simulink model "Quadrotor"  (R2022b)
settings: Solver=FixedStepAuto  StartTime=0.0  StopTime=1000  FixedStep=0.0005  RelTol=1e-3
model workspace (MAT data in the model file):
  b = 0.000142
  g = 9.8
  m = 1
undefined symbols (not defined in the file): Pitch, Roll, X, Y, Yaw, Z
libraries: simulink x12, slpidlib x9, sharedtransform x1, uavutilslib x1, aerolibanim x1
(part 3 of 3)

== system Quadrotor/Attitude Loop(LADRC)/LADRC/TD ==
  v0 : Inport
  Constant : Constant  Value=r
  Constant1 : Constant  Value=0.05
  Gain : Gain  Gain=h
  Gain1 : Gain  Gain=h
  MATLAB Function : MATLAB Function  TreatAsAtomicUnit=on
  Sum : Sum  Inputs=+-|
  Sum1 : Sum  Inputs=++|
  Sum2 : Sum  Inputs=++|
  Unit Delay : UnitDelay  SampleTime=-1  HasFrameUpgradeWarning=on
  Unit Delay1 : UnitDelay  SampleTime=-1  HasFrameUpgradeWarning=on
  v1 : Outport
  v2 : Outport  Port=2
  wires:
  v0/1 -> Sum/2
  Unit Delay/1 -> Sum1/1, Sum/1  "v1(k"
  Unit Delay1/1 -> Sum2/1, MATLAB Function/2(v1), Gain/1  "v2(k)"
  Gain/1 -> Sum1/2
  Sum1/1 -> v1/1, Unit Delay/1  "v1(k+1)"
  Gain1/1 -> Sum2/2
  Sum2/1 -> v2/1, Unit Delay1/1  "v2(k+1)"
  MATLAB Function/1(y) -> Gain1/1
  Constant/1 -> MATLAB Function/3(r)
  Sum/1 -> MATLAB Function/1(delta)

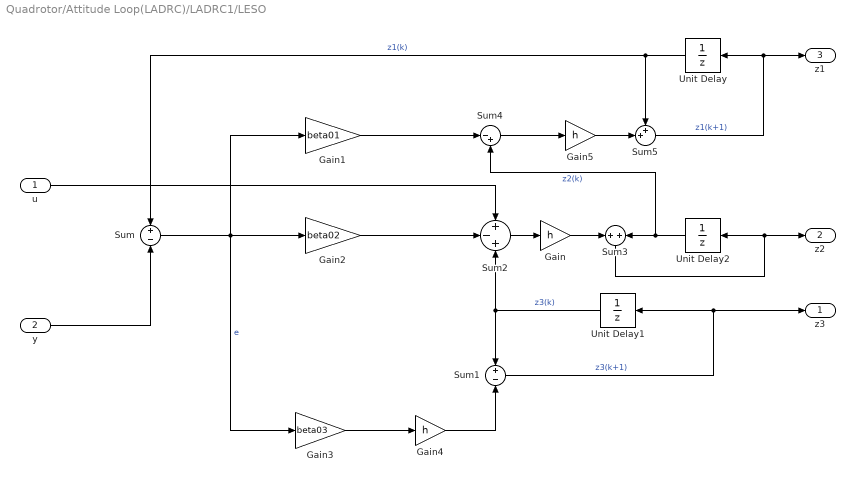
== system Quadrotor/Attitude Loop(LADRC)/LADRC1/LESO ==
  u : Inport
  y : Inport  Port=2
  Gain : Gain  Gain=h
  Gain1 : Gain  Gain=beta01
  Gain2 : Gain  Gain=beta02
  Gain3 : Gain  Gain=beta03
  Gain4 : Gain  Gain=h
  Gain5 : Gain  Gain=h
  Sum : Sum  Inputs=+|-
  Sum1 : Sum  Inputs=+-
  Sum2 : Sum  Inputs=+-+
  Sum3 : Sum
  Sum4 : Sum  Inputs=|-+
  Sum5 : Sum  Inputs=++|
  Unit Delay : UnitDelay  SampleTime=-1  HasFrameUpgradeWarning=on
  Unit Delay1 : UnitDelay  SampleTime=-1  HasFrameUpgradeWarning=on
  Unit Delay2 : UnitDelay  SampleTime=-1  HasFrameUpgradeWarning=on
  z3 : Outport
  z2 : Outport  Port=2
  z1 : Outport  Port=3
  wires:
  y/1 -> Sum/2
  Unit Delay/1 -> Sum/1, Sum5/1  "z1(k)"
  Unit Delay1/1 -> Sum2/3, Sum1/1  "z3(k)"
  Sum/1 -> Gain3/1, Gain1/1, Gain2/1  "e"
  Gain3/1 -> Gain4/1
  Gain4/1 -> Sum1/2
  Sum1/1 -> z3/1, Unit Delay1/1  "z3(k+1)"
  Gain2/1 -> Sum2/2
  Sum2/1 -> Gain/1
  Gain/1 -> Sum3/1
  Unit Delay2/1 -> Sum4/2, Sum3/2  "z2(k)"
  Sum3/1 -> Unit Delay2/1, z2/1
  Gain1/1 -> Sum4/1
  Sum4/1 -> Gain5/1
  Gain5/1 -> Sum5/2
  Sum5/1 -> Unit Delay/1, z1/1  "z1(k+1)"
  u/1 -> Sum2/1

== system Quadrotor/Attitude Loop(LADRC)/LADRC1/LSEF ==
  e1 : Inport
  e2 : Inport  Port=2
  Sum : Sum  Inputs=+-
  kp1 : Gain  Gain=kp1
  kp2 : Gain  Gain=kp2
  u0 : Outport
  wires:
  e1/1 -> kp1/1
  e2/1 -> kp2/1
  kp1/1 -> Sum/1
  kp2/1 -> Sum/2
  Sum/1 -> u0/1

== system Quadrotor/Attitude Loop(LADRC)/P&R/Pitch_LADRC ==
  v0 : Inport
  y : Inport  Port=2
  LESO : Subsystem
      settings: PortSchema="{\"entries\":[{\"content\":{\"sides\":[{\"content\":{\"connectorIds\":[]},\"type\":\"ConnectorPlacement.EquallySpacedRectSide\",\"uuid\":\"29853f4c-4dde-4de5-ade1-1dc0b5f537cd\"},{\"content\":{\"connectorIds\":[\"Out1\",\"Out2\",\"Out3\"],\"side\":\"RIGHT\"},\"type\":\"ConnectorPlacement.EquallySpacedRectSide\",\"uuid\":\"f82e0ac0-07eb-4296-b691-afdbd004b121\"},{\"content\":{\"connectorIds\":[\"In1\"],\"side\":\"TOP\"},\"type\":\"ConnectorPlacement.EquallySpacedRectSide\",\"uuid\":\"058c0543-22b7-4f39-8eab-a4fe87266d7e\"},{\"content\":{\"connectorIds\":[\"In2\"],\"side\":\"BOTTOM\"},\"type\":\"ConnectorPlacement.EquallySpacedRectSide\",\"uuid\":\"5206ee30-69dc-4d41-920c-ca25503196a3\"}]},\"type\":\"ConnectorPlacement.EquallySpacedConnector\",\"uuid\":\"8c454db7-eb5f-43d2-ac3f-1394779a05da\"}],\"packageUris\":[\"http://schema.mathworks.com/mf0/Connector/19700101\"],\"version\":\"1.0\"}"
  LSEF : Subsystem
  Sum : Sum  Inputs=|+-
  Sum1 : Sum  Inputs=|+-
  Sum2 : Sum  Inputs=|+-
  TD : Subsystem
  b1 : Gain  Gain=b
  b2 : Gain  Gain=1/b
  u : Outport
  wires:
  LESO/3(z1) -> Sum/2  "z1"
  LSEF/1(u0) -> Sum2/1
  Sum/1 -> LSEF/1(e1)  "e1"
  LESO/1(z3) -> Sum2/2
  Sum2/1 -> b2/1  "e1"
  b2/1 -> b1/1, u/1
  y/1 -> LESO/2(y)
  TD/1(v1) -> Sum/1
  v0/1 -> TD/1(v0)
  TD/2(v2) -> Sum1/1
  Sum1/1 -> LSEF/2(e2)  "e2"
  LESO/2(z2) -> Sum1/2  "z2"
  b1/1 -> LESO/1(u)

== system Quadrotor/Attitude Loop(LADRC)/P&R/Roll_LADRC ==
  v0 : Inport
  y : Inport  Port=2
  LESO : Subsystem
      settings: PortSchema="{\"entries\":[{\"content\":{\"sides\":[{\"content\":{\"connectorIds\":[]},\"type\":\"ConnectorPlacement.EquallySpacedRectSide\",\"uuid\":\"29853f4c-4dde-4de5-ade1-1dc0b5f537cd\"},{\"content\":{\"connectorIds\":[\"Out1\",\"Out2\",\"Out3\"],\"side\":\"RIGHT\"},\"type\":\"ConnectorPlacement.EquallySpacedRectSide\",\"uuid\":\"f82e0ac0-07eb-4296-b691-afdbd004b121\"},{\"content\":{\"connectorIds\":[\"In1\"],\"side\":\"TOP\"},\"type\":\"ConnectorPlacement.EquallySpacedRectSide\",\"uuid\":\"058c0543-22b7-4f39-8eab-a4fe87266d7e\"},{\"content\":{\"connectorIds\":[\"In2\"],\"side\":\"BOTTOM\"},\"type\":\"ConnectorPlacement.EquallySpacedRectSide\",\"uuid\":\"5206ee30-69dc-4d41-920c-ca25503196a3\"}]},\"type\":\"ConnectorPlacement.EquallySpacedConnector\",\"uuid\":\"8c454db7-eb5f-43d2-ac3f-1394779a05da\"}],\"packageUris\":[\"http://schema.mathworks.com/mf0/Connector/19700101\"],\"version\":\"1.0\"}"
  LSEF : Subsystem
  Sum : Sum  Inputs=|+-
  Sum1 : Sum  Inputs=|+-
  Sum2 : Sum  Inputs=|+-
  TD : Subsystem
  b1 : Gain  Gain=b
  b2 : Gain  Gain=1/b
  u : Outport
  wires:
  LESO/3(z1) -> Sum/2  "z1"
  LSEF/1(u0) -> Sum2/1
  Sum/1 -> LSEF/1(e1)  "e1"
  LESO/1(z3) -> Sum2/2
  Sum2/1 -> b2/1  "e1"
  b2/1 -> b1/1, u/1
  y/1 -> LESO/2(y)
  TD/1(v1) -> Sum/1
  v0/1 -> TD/1(v0)
  TD/2(v2) -> Sum1/1
  Sum1/1 -> LSEF/2(e2)  "e2"
  LESO/2(z2) -> Sum1/2  "z2"
  b1/1 -> LESO/1(u)

== system Quadrotor/Attitude Loop(LADRC)/yaw/Yaw_LADRC ==
  v0 : Inport
  y : Inport  Port=2
  LESO : Subsystem
      settings: PortSchema="{\"entries\":[{\"content\":{\"sides\":[{\"content\":{\"connectorIds\":[]},\"type\":\"ConnectorPlacement.EquallySpacedRectSide\",\"uuid\":\"29853f4c-4dde-4de5-ade1-1dc0b5f537cd\"},{\"content\":{\"connectorIds\":[\"Out1\",\"Out2\",\"Out3\"],\"side\":\"RIGHT\"},\"type\":\"ConnectorPlacement.EquallySpacedRectSide\",\"uuid\":\"f82e0ac0-07eb-4296-b691-afdbd004b121\"},{\"content\":{\"connectorIds\":[\"In1\"],\"side\":\"TOP\"},\"type\":\"ConnectorPlacement.EquallySpacedRectSide\",\"uuid\":\"058c0543-22b7-4f39-8eab-a4fe87266d7e\"},{\"content\":{\"connectorIds\":[\"In2\"],\"side\":\"BOTTOM\"},\"type\":\"ConnectorPlacement.EquallySpacedRectSide\",\"uuid\":\"5206ee30-69dc-4d41-920c-ca25503196a3\"}]},\"type\":\"ConnectorPlacement.EquallySpacedConnector\",\"uuid\":\"8c454db7-eb5f-43d2-ac3f-1394779a05da\"}],\"packageUris\":[\"http://schema.mathworks.com/mf0/Connector/19700101\"],\"version\":\"1.0\"}"
  LSEF : Subsystem
  Sum : Sum  Inputs=|+-
  Sum1 : Sum  Inputs=|+-
  Sum2 : Sum  Inputs=|+-
  TD : Subsystem
  b1 : Gain  Gain=b
  b2 : Gain  Gain=1/b
  u : Outport
  wires:
  LESO/3(z1) -> Sum/2  "z1"
  LSEF/1(u0) -> Sum2/1
  Sum/1 -> LSEF/1(e1)  "e1"
  LESO/1(z3) -> Sum2/2
  Sum2/1 -> b2/1  "e3"
  b2/1 -> b1/1, u/1
  y/1 -> LESO/2(y)
  TD/1(v1) -> Sum/1
  v0/1 -> TD/1(v0)
  TD/2(v2) -> Sum1/1
  Sum1/1 -> LSEF/2(e2)  "e2"
  LESO/2(z2) -> Sum1/2  "z2"
  b1/1 -> LESO/1(u)

== system Quadrotor/Demand_LADRC/generate/butterfly ==
  Bus Creator : BusCreator  Inputs=4
  Gain : Gain
  Gain1 : Gain
  MATLAB Function : MATLAB Function  TreatAsAtomicUnit=on
  MATLAB Function1 : MATLAB Function  TreatAsAtomicUnit=on
  Ramp : simulink/Sources/Ramp  slope=1  start=0  InitialOutput=0
  Ramp1 : simulink/Sources/Ramp  slope=1  start=0  InitialOutput=0
  yaw* : Constant  Value=0
  z* : Constant  Value=5
  Out1 : Outport
  wires:
  Ramp1/1 -> MATLAB Function1/1(t)
  z*/1 -> Bus Creator/3
  Ramp/1 -> MATLAB Function/1(t)
  yaw*/1 -> Bus Creator/4
  Gain/1 -> Bus Creator/1
  Gain1/1 -> Bus Creator/2
  Bus Creator/1 -> Out1/1
  MATLAB Function/1(x) -> Gain/1
  MATLAB Function1/1(y) -> Gain1/1

== system Quadrotor/Demand_LADRC/generate/circle 500 ==
  Bus Creator : BusCreator  Inputs=4
  x* : Sin  SineType=Sample based  Frequency=2*pi*.003  Phase=-pi/2  SampleTime=0.0005
  y* : Sin  SineType=Sample based  Frequency=2*pi*.003  SampleTime=0.0005
  yaw* : Constant  Value=0
  z* : Constant  Value=3
  Out1 : Outport
  wires:
  Bus Creator/1 -> Out1/1
  z*/1 -> Bus Creator/3
  y*/1 -> Bus Creator/2
  yaw*/1 -> Bus Creator/4
  x*/1 -> Bus Creator/1

== system Quadrotor/Demand_LADRC/generate/ramp 30 ==
  Bus Creator : BusCreator  Inputs=4
  x_s : Constant  Value=0
  y_s : simulink/Sources/Ramp  slope=0.2  start=0  InitialOutput=0
  yaw_s : Constant  Value=0
  z_s3 : simulink/Sources/Ramp  slope=0.1  start=0  InitialOutput=0
  Out1 : Outport
  wires:
  z_s3/1 -> Bus Creator/3
  Bus Creator/1 -> Out1/1
  x_s/1 -> Bus Creator/1
  y_s/1 -> Bus Creator/2
  yaw_s/1 -> Bus Creator/4

== system Quadrotor/Demand_LADRC/generate/screw 600 ==
  Bus Creator1 : BusCreator  Inputs=4
  x*2 : Sin  Frequency=2*pi*.003  Phase=-pi/2  SampleTime=0
  y*2 : Sin  Frequency=2*pi*.003  SampleTime=0
  yaw*2 : Constant  Value=0.2
  z_s4 : simulink/Sources/Ramp  slope=0.005  start=0  InitialOutput=0
  Out1 : Outport
  wires:
  x*2/1 -> Bus Creator1/1
  z_s4/1 -> Bus Creator1/3
  Bus Creator1/1 -> Out1/1
  y*2/1 -> Bus Creator1/2
  yaw*2/1 -> Bus Creator1/4

== system Quadrotor/Demand_LADRC/generate/steady1 ==
  Bus Creator2 : BusCreator  Inputs=4
  x_s2 : Constant
  y_s1 : Constant
  y_s2 : Constant
  yaw_s2 : Constant  Value=0
  Out1 : Outport
  wires:
  y_s2/1 -> Bus Creator2/2
  yaw_s2/1 -> Bus Creator2/4
  Bus Creator2/1 -> Out1/1
  y_s1/1 -> Bus Creator2/3
  x_s2/1 -> Bus Creator2/1

== system Quadrotor/Demand_LADRC/generate/up 30 ==
  Bus Creator2 : BusCreator  Inputs=4
  x_s2 : Constant  Value=0
  y_s2 : Constant  Value=0
  yaw_s2 : Constant  Value=0
  z_s2 : simulink/Sources/Ramp  slope=0.2  start=0  InitialOutput=0
  Out1 : Outport
  wires:
  y_s2/1 -> Bus Creator2/2
  yaw_s2/1 -> Bus Creator2/4
  Bus Creator2/1 -> Out1/1
  z_s2/1 -> Bus Creator2/3
  x_s2/1 -> Bus Creator2/1

== system Quadrotor/Demand_PID/generate/butterfly ==
  Bus Creator : BusCreator  Inputs=4
  Gain : Gain
  Gain1 : Gain
  MATLAB Function : MATLAB Function  TreatAsAtomicUnit=on
  MATLAB Function1 : MATLAB Function  TreatAsAtomicUnit=on
  Ramp : simulink/Sources/Ramp  slope=1  start=0  InitialOutput=0
  Ramp1 : simulink/Sources/Ramp  slope=1  start=0  InitialOutput=0
  yaw* : Constant  Value=0
  z* : Constant  Value=5
  Out1 : Outport
  wires:
  Ramp1/1 -> MATLAB Function1/1(t)
  z*/1 -> Bus Creator/3
  Ramp/1 -> MATLAB Function/1(t)
  yaw*/1 -> Bus Creator/4
  Gain/1 -> Bus Creator/1
  Gain1/1 -> Bus Creator/2
  Bus Creator/1 -> Out1/1
  MATLAB Function/1(x) -> Gain/1
  MATLAB Function1/1(y) -> Gain1/1

== system Quadrotor/Demand_PID/generate/circle 500 ==
  Bus Creator : BusCreator  Inputs=4
  x* : Sin  Frequency=2*pi*.003  Phase=-pi/2  SampleTime=0
  y* : Sin  Frequency=2*pi*.003  SampleTime=0
  yaw* : Constant  Value=0
  z* : Constant  Value=3
  Out1 : Outport
  wires:
  Bus Creator/1 -> Out1/1
  z*/1 -> Bus Creator/3
  y*/1 -> Bus Creator/2
  yaw*/1 -> Bus Creator/4
  x*/1 -> Bus Creator/1

== system Quadrotor/Demand_PID/generate/ramp 30 ==
  Bus Creator : BusCreator  Inputs=4
  x_s : Constant  Value=0
  y_s : simulink/Sources/Ramp  slope=0.2  start=0  InitialOutput=0
  yaw_s : Constant  Value=0
  z_s3 : simulink/Sources/Ramp  slope=0.1  start=0  InitialOutput=0
  Out1 : Outport
  wires:
  z_s3/1 -> Bus Creator/3
  Bus Creator/1 -> Out1/1
  x_s/1 -> Bus Creator/1
  y_s/1 -> Bus Creator/2
  yaw_s/1 -> Bus Creator/4

== system Quadrotor/Demand_PID/generate/screw 600 ==
  Bus Creator1 : BusCreator  Inputs=4
  x*2 : Sin  Frequency=2*pi*.003  Phase=-pi/2  SampleTime=0
  y*2 : Sin  Frequency=2*pi*.003  SampleTime=0
  yaw*2 : Constant  Value=0
  z_s4 : simulink/Sources/Ramp  slope=0.005  start=0  InitialOutput=0
  Out1 : Outport
  wires:
  yaw*2/1 -> Bus Creator1/4
  x*2/1 -> Bus Creator1/1
  z_s4/1 -> Bus Creator1/3
  Bus Creator1/1 -> Out1/1
  y*2/1 -> Bus Creator1/2

== system Quadrotor/Demand_PID/generate/steady1 ==
  Bus Creator2 : BusCreator  Inputs=4
  x_s2 : Constant
  y_s1 : Constant
  y_s2 : Constant
  yaw_s2 : Constant  Value=0
  Out1 : Outport
  wires:
  y_s2/1 -> Bus Creator2/2
  yaw_s2/1 -> Bus Creator2/4
  Bus Creator2/1 -> Out1/1
  y_s1/1 -> Bus Creator2/3
  x_s2/1 -> Bus Creator2/1

== system Quadrotor/Demand_PID/generate/up 30 ==
  Bus Creator2 : BusCreator  Inputs=4
  x_s2 : Constant  Value=0
  y_s2 : Constant  Value=0
  yaw_s2 : Constant  Value=0
  z_s2 : simulink/Sources/Ramp  slope=0.2  start=0  InitialOutput=0
  Out1 : Outport
  wires:
  y_s2/1 -> Bus Creator2/2
  yaw_s2/1 -> Bus Creator2/4
  Bus Creator2/1 -> Out1/1
  z_s2/1 -> Bus Creator2/3
  x_s2/1 -> Bus Creator2/1

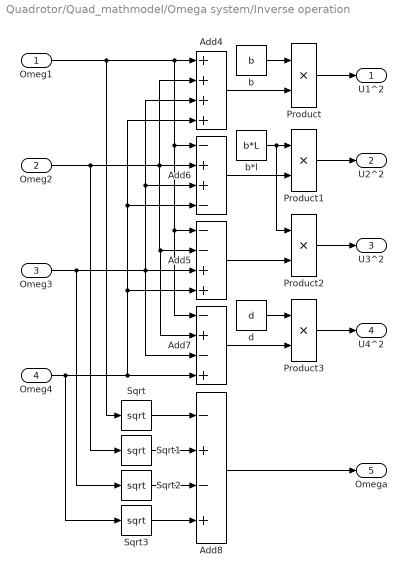
== system Quadrotor/Quad_mathmodel/Omega system/Inverse operation ==
  Omeg1 : Inport
  Omeg2 : Inport  Port=2
  Omeg3 : Inport  Port=3
  Omeg4 : Inport  Port=4
  Add4 : Sum  Inputs=++++
  Add5 : Sum  Inputs=--++
  Add6 : Sum  Inputs=-++-
  Add7 : Sum  Inputs=-+-+
  Add8 : Sum  Inputs=-+-+
  Product{,1..3} (4 alike) : Product
  Sqrt{,1..3} (4 alike) : Sqrt
  b : Constant  Value=b
  b*l : Constant  Value=b*L
  d : Constant  Value=d
  U1^2 : Outport
  U2^2 : Outport  Port=2
  U3^2 : Outport  Port=3
  U4^2 : Outport  Port=4
  Omega : Outport  Port=5
  wires:
  Omeg1/1 -> Add7/1, Add5/1, Add6/1, Add4/1, Sqrt/1
  Product2/1 -> U3^2/1
  Add5/1 -> Product2/2
  Add8/1 -> Omega/1
  Product3/1 -> U4^2/1
  Add6/1 -> Product1/2
  b/1 -> Product/1
  Add4/1 -> Product/2
  Omeg4/1 -> Sqrt3/1, Add5/4, Add6/4, Add4/4, Add7/4
  b*l/1 -> Product2/1, Product1/1
  Product1/1 -> U2^2/1
  d/1 -> Product3/1
  Sqrt/1 -> Add8/1
  Sqrt3/1 -> Add8/4
  Omeg3/1 -> Sqrt2/1, Add7/3, Add6/3, Add4/3, Add5/3
  Omeg2/1 -> Sqrt1/1, Add7/2, Add5/2, Add4/2, Add6/2
  Sqrt1/1 -> Add8/2
  Add7/1 -> Product3/2
  Sqrt2/1 -> Add8/3
  Product/1 -> U1^2/1

== system Quadrotor/Quad_mathmodel/Omega system/operation ==
  U1 : Inport
  U2 : Inport  Port=2
  U3 : Inport  Port=3
  U4 : Inport  Port=4
  4*b : Constant  Value=4*b
  4*b*l : Constant  Value=4*b*L
  4*d : Constant  Value=4*d
  Add : Sum  Inputs=+---
  Add1 : Sum  Inputs=++-+
  Add2 : Sum  Inputs=+++-
  Add3 : Sum  Inputs=+-++
  Divide{,1..3} (4 alike) : Product  Inputs=*/
  Omeg1 : Outport
  Omeg2 : Outport  Port=2
  Omeg3 : Outport  Port=3
  Omeg4 : Outport  Port=4
  wires:
  U1/1 -> Divide/1
  4*b*l/1 -> Divide2/2, Divide1/2
  U3/1 -> Divide2/1
  Divide3/1 -> Add3/4, Add/4, Add1/4, Add2/4
  U2/1 -> Divide1/1
  Divide1/1 -> Add3/2, Add2/2, Add1/2, Add/2
  Add1/1 -> Omeg2/1
  4*d/1 -> Divide3/2
  Divide2/1 -> Add2/3, Add3/3, Add1/3, Add/3
  Divide/1 -> Add/1, Add1/1, Add2/1, Add3/1
  4*b/1 -> Divide/2
  U4/1 -> Divide3/1
  Add3/1 -> Omeg4/1
  Add2/1 -> Omeg3/1
  Add/1 -> Omeg1/1

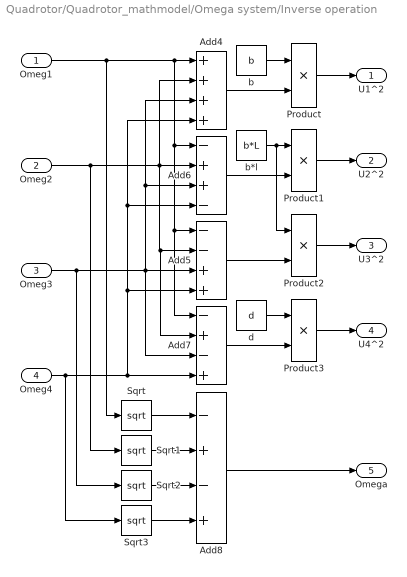
== system Quadrotor/Quadrotor_mathmodel/Omega system/Inverse operation ==
  Omeg1 : Inport
  Omeg2 : Inport  Port=2
  Omeg3 : Inport  Port=3
  Omeg4 : Inport  Port=4
  Add4 : Sum  Inputs=++++
  Add5 : Sum  Inputs=--++
  Add6 : Sum  Inputs=-++-
  Add7 : Sum  Inputs=-+-+
  Add8 : Sum  Inputs=-+-+
  Product{,1..3} (4 alike) : Product
  Sqrt{,1..3} (4 alike) : Sqrt
  b : Constant  Value=b
  b*l : Constant  Value=b*L
  d : Constant  Value=d
  U1^2 : Outport
  U2^2 : Outport  Port=2
  U3^2 : Outport  Port=3
  U4^2 : Outport  Port=4
  Omega : Outport  Port=5
  wires:
  Omeg1/1 -> Add7/1, Add5/1, Add6/1, Add4/1, Sqrt/1
  Product2/1 -> U3^2/1
  Add5/1 -> Product2/2
  Add8/1 -> Omega/1
  Product3/1 -> U4^2/1
  Add6/1 -> Product1/2
  b/1 -> Product/1
  Add4/1 -> Product/2
  Omeg4/1 -> Sqrt3/1, Add5/4, Add6/4, Add4/4, Add7/4
  b*l/1 -> Product2/1, Product1/1
  Product1/1 -> U2^2/1
  d/1 -> Product3/1
  Sqrt/1 -> Add8/1
  Sqrt3/1 -> Add8/4
  Omeg3/1 -> Sqrt2/1, Add7/3, Add6/3, Add4/3, Add5/3
  Omeg2/1 -> Sqrt1/1, Add7/2, Add5/2, Add4/2, Add6/2
  Sqrt1/1 -> Add8/2
  Add7/1 -> Product3/2
  Sqrt2/1 -> Add8/3
  Product/1 -> U1^2/1

== system Quadrotor/Quadrotor_mathmodel/Omega system/operation ==
  U1 : Inport
  U2 : Inport  Port=2
  U3 : Inport  Port=3
  U4 : Inport  Port=4
  4*b : Constant  Value=4*b
  4*b*l : Constant  Value=4*b*L
  4*d : Constant  Value=4*d
  Add : Sum  Inputs=+---
  Add1 : Sum  Inputs=++-+
  Add2 : Sum  Inputs=+++-
  Add3 : Sum  Inputs=+-++
  Divide{,1..3} (4 alike) : Product  Inputs=*/
  Omeg1 : Outport
  Omeg2 : Outport  Port=2
  Omeg3 : Outport  Port=3
  Omeg4 : Outport  Port=4
  wires:
  U1/1 -> Divide/1
  4*b*l/1 -> Divide2/2, Divide1/2
  U3/1 -> Divide2/1
  Divide3/1 -> Add3/4, Add/4, Add1/4, Add2/4
  U2/1 -> Divide1/1
  Divide1/1 -> Add3/2, Add2/2, Add1/2, Add/2
  Add1/1 -> Omeg2/1
  4*d/1 -> Divide3/2
  Divide2/1 -> Add2/3, Add3/3, Add1/3, Add/3
  Divide/1 -> Add/1, Add1/1, Add2/1, Add3/1
  4*b/1 -> Divide/2
  U4/1 -> Divide3/1
  Add3/1 -> Omeg4/1
  Add2/1 -> Omeg3/1
  Add/1 -> Omeg1/1

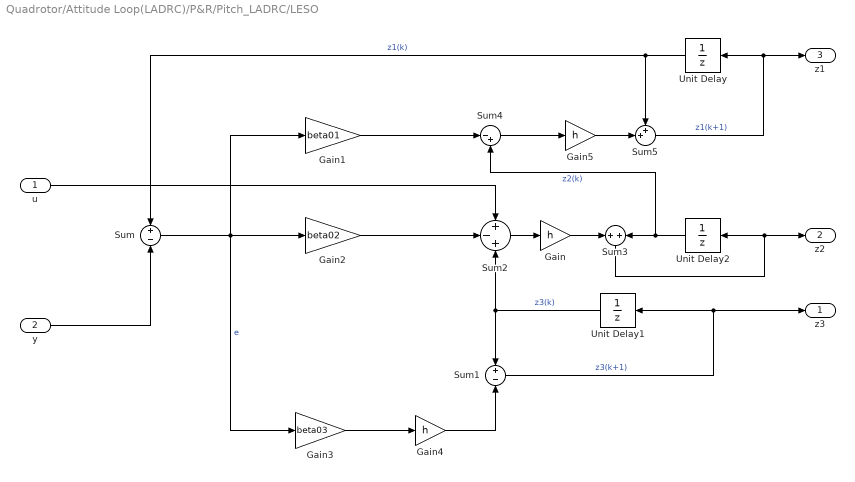
== system Quadrotor/Attitude Loop(LADRC)/P&R/Pitch_LADRC/LESO ==
  u : Inport
  y : Inport  Port=2
  Gain : Gain  Gain=h
  Gain1 : Gain  Gain=beta01
  Gain2 : Gain  Gain=beta02
  Gain3 : Gain  Gain=beta03
  Gain4 : Gain  Gain=h
  Gain5 : Gain  Gain=h
  Sum : Sum  Inputs=+|-
  Sum1 : Sum  Inputs=+-
  Sum2 : Sum  Inputs=+-+
  Sum3 : Sum
  Sum4 : Sum  Inputs=|-+
  Sum5 : Sum  Inputs=++|
  Unit Delay : UnitDelay  SampleTime=-1  HasFrameUpgradeWarning=on
  Unit Delay1 : UnitDelay  SampleTime=-1  HasFrameUpgradeWarning=on
  Unit Delay2 : UnitDelay  SampleTime=-1  HasFrameUpgradeWarning=on
  z3 : Outport
  z2 : Outport  Port=2
  z1 : Outport  Port=3
  wires:
  y/1 -> Sum/2
  Unit Delay/1 -> Sum/1, Sum5/1  "z1(k)"
  Unit Delay1/1 -> Sum2/3, Sum1/1  "z3(k)"
  Sum/1 -> Gain3/1, Gain1/1, Gain2/1  "e"
  Gain3/1 -> Gain4/1
  Gain4/1 -> Sum1/2
  Sum1/1 -> z3/1, Unit Delay1/1  "z3(k+1)"
  Gain2/1 -> Sum2/2
  Sum2/1 -> Gain/1
  Gain/1 -> Sum3/1
  Unit Delay2/1 -> Sum4/2, Sum3/2  "z2(k)"
  Sum3/1 -> Unit Delay2/1, z2/1
  Gain1/1 -> Sum4/1
  Sum4/1 -> Gain5/1
  Gain5/1 -> Sum5/2
  Sum5/1 -> Unit Delay/1, z1/1  "z1(k+1)"
  u/1 -> Sum2/1

== system Quadrotor/Attitude Loop(LADRC)/P&R/Pitch_LADRC/LSEF ==
  e1 : Inport
  e2 : Inport  Port=2
  Sum : Sum
  kp1 : Gain  Gain=kp1
  kp2 : Gain  Gain=kp2
  u0 : Outport
  wires:
  e1/1 -> kp1/1
  e2/1 -> kp2/1
  kp1/1 -> Sum/1
  kp2/1 -> Sum/2
  Sum/1 -> u0/1

== system Quadrotor/Attitude Loop(LADRC)/P&R/Pitch_LADRC/TD ==
  v0 : Inport
  Constant : Constant  Value=r
  Constant1 : Constant  Value=0.05
  Gain : Gain  Gain=h
  Gain1 : Gain  Gain=h
  MATLAB Function : MATLAB Function  TreatAsAtomicUnit=on
  Sum : Sum  Inputs=+-|
  Sum1 : Sum  Inputs=++|
  Sum2 : Sum  Inputs=++|
  Unit Delay : UnitDelay  SampleTime=-1  HasFrameUpgradeWarning=on
  Unit Delay1 : UnitDelay  SampleTime=-1  HasFrameUpgradeWarning=on
  v1 : Outport
  v2 : Outport  Port=2
  wires:
  v0/1 -> Sum/2
  Unit Delay/1 -> Sum1/1, Sum/1  "v1(k"
  Unit Delay1/1 -> Sum2/1, MATLAB Function/2(v1), Gain/1  "v2(k)"
  Gain/1 -> Sum1/2
  Sum1/1 -> v1/1, Unit Delay/1  "v1(k+1)"
  Gain1/1 -> Sum2/2
  Sum2/1 -> v2/1, Unit Delay1/1  "v2(k+1)"
  MATLAB Function/1(y) -> Gain1/1
  Constant/1 -> MATLAB Function/3(r)
  Sum/1 -> MATLAB Function/1(delta)

== system Quadrotor/Attitude Loop(LADRC)/P&R/Roll_LADRC/LESO ==
  u : Inport
  y : Inport  Port=2
  Gain : Gain  Gain=h
  Gain1 : Gain  Gain=beta01
  Gain2 : Gain  Gain=beta02
  Gain3 : Gain  Gain=beta03
  Gain4 : Gain  Gain=h
  Gain5 : Gain  Gain=h
  Sum : Sum  Inputs=+|-
  Sum1 : Sum  Inputs=+-
  Sum2 : Sum  Inputs=+-+
  Sum3 : Sum
  Sum4 : Sum  Inputs=|-+
  Sum5 : Sum  Inputs=++|
  Unit Delay : UnitDelay  SampleTime=-1  HasFrameUpgradeWarning=on
  Unit Delay1 : UnitDelay  SampleTime=-1  HasFrameUpgradeWarning=on
  Unit Delay2 : UnitDelay  SampleTime=-1  HasFrameUpgradeWarning=on
  z3 : Outport
  z2 : Outport  Port=2
  z1 : Outport  Port=3
  wires:
  y/1 -> Sum/2
  Unit Delay/1 -> Sum/1, Sum5/1  "z1(k)"
  Unit Delay1/1 -> Sum2/3, Sum1/1  "z3(k)"
  Sum/1 -> Gain3/1, Gain1/1, Gain2/1  "e"
  Gain3/1 -> Gain4/1
  Gain4/1 -> Sum1/2
  Sum1/1 -> z3/1, Unit Delay1/1  "z3(k+1)"
  Gain2/1 -> Sum2/2
  Sum2/1 -> Gain/1
  Gain/1 -> Sum3/1
  Unit Delay2/1 -> Sum4/2, Sum3/2  "z2(k)"
  Sum3/1 -> Unit Delay2/1, z2/1
  Gain1/1 -> Sum4/1
  Sum4/1 -> Gain5/1
  Gain5/1 -> Sum5/2
  Sum5/1 -> Unit Delay/1, z1/1  "z1(k+1)"
  u/1 -> Sum2/1

== system Quadrotor/Attitude Loop(LADRC)/P&R/Roll_LADRC/LSEF ==
  e1 : Inport
  e2 : Inport  Port=2
  Sum : Sum
  kp1 : Gain  Gain=kp1
  kp2 : Gain  Gain=kp2
  u0 : Outport
  wires:
  e1/1 -> kp1/1
  e2/1 -> kp2/1
  kp1/1 -> Sum/1
  kp2/1 -> Sum/2
  Sum/1 -> u0/1

== system Quadrotor/Attitude Loop(LADRC)/P&R/Roll_LADRC/TD ==
  v0 : Inport
  Constant : Constant  Value=r
  Constant1 : Constant  Value=0.05
  Gain : Gain  Gain=h
  Gain1 : Gain  Gain=h
  MATLAB Function : MATLAB Function  TreatAsAtomicUnit=on
  Sum : Sum  Inputs=+-|
  Sum1 : Sum  Inputs=++|
  Sum2 : Sum  Inputs=++|
  Unit Delay : UnitDelay  SampleTime=-1  HasFrameUpgradeWarning=on
  Unit Delay1 : UnitDelay  SampleTime=-1  HasFrameUpgradeWarning=on
  v1 : Outport
  v2 : Outport  Port=2
  wires:
  v0/1 -> Sum/2
  Unit Delay/1 -> Sum1/1, Sum/1  "v1(k"
  Unit Delay1/1 -> Sum2/1, MATLAB Function/2(v1), Gain/1  "v2(k)"
  Gain/1 -> Sum1/2
  Sum1/1 -> v1/1, Unit Delay/1  "v1(k+1)"
  Gain1/1 -> Sum2/2
  Sum2/1 -> v2/1, Unit Delay1/1  "v2(k+1)"
  MATLAB Function/1(y) -> Gain1/1
  Constant/1 -> MATLAB Function/3(r)
  Sum/1 -> MATLAB Function/1(delta)

== system Quadrotor/Attitude Loop(LADRC)/yaw/Yaw_LADRC/LESO ==
  u : Inport
  y : Inport  Port=2
  Gain : Gain  Gain=h
  Gain1 : Gain  Gain=beta01
  Gain2 : Gain  Gain=beta02
  Gain3 : Gain  Gain=beta03
  Gain4 : Gain  Gain=h
  Gain5 : Gain  Gain=h
  Sum : Sum  Inputs=+|-
  Sum1 : Sum  Inputs=+-
  Sum2 : Sum  Inputs=+-+
  Sum3 : Sum
  Sum4 : Sum  Inputs=|-+
  Sum5 : Sum  Inputs=++|
  Unit Delay : UnitDelay  SampleTime=-1  HasFrameUpgradeWarning=on
  Unit Delay1 : UnitDelay  SampleTime=-1  HasFrameUpgradeWarning=on
  Unit Delay2 : UnitDelay  SampleTime=-1  HasFrameUpgradeWarning=on
  z3 : Outport
  z2 : Outport  Port=2
  z1 : Outport  Port=3
  wires:
  y/1 -> Sum/2
  Unit Delay/1 -> Sum/1, Sum5/1  "z1(k)"
  Unit Delay1/1 -> Sum2/3, Sum1/1  "z3(k)"
  Sum/1 -> Gain3/1, Gain1/1, Gain2/1  "e"
  Gain3/1 -> Gain4/1
  Gain4/1 -> Sum1/2
  Sum1/1 -> z3/1, Unit Delay1/1  "z3(k+1)"
  Gain2/1 -> Sum2/2
  Sum2/1 -> Gain/1
  Gain/1 -> Sum3/1
  Unit Delay2/1 -> Sum4/2, Sum3/2  "z2(k)"
  Sum3/1 -> Unit Delay2/1, z2/1
  Gain1/1 -> Sum4/1
  Sum4/1 -> Gain5/1
  Gain5/1 -> Sum5/2
  Sum5/1 -> Unit Delay/1, z1/1  "z1(k+1)"
  u/1 -> Sum2/1

== system Quadrotor/Attitude Loop(LADRC)/yaw/Yaw_LADRC/LSEF ==
  e1 : Inport
  e2 : Inport  Port=2
  Sum : Sum
  kp1 : Gain  Gain=kp1
  kp2 : Gain  Gain=kp2
  u0 : Outport
  wires:
  e1/1 -> kp1/1
  e2/1 -> kp2/1
  kp1/1 -> Sum/1
  kp2/1 -> Sum/2
  Sum/1 -> u0/1

== system Quadrotor/Attitude Loop(LADRC)/yaw/Yaw_LADRC/TD ==
  v0 : Inport
  Constant : Constant  Value=r
  Constant1 : Constant  Value=0.05
  Gain : Gain  Gain=h
  Gain1 : Gain  Gain=h
  MATLAB Function : MATLAB Function  TreatAsAtomicUnit=on
  Sum : Sum  Inputs=+-|
  Sum1 : Sum  Inputs=++|
  Sum2 : Sum  Inputs=++|
  Unit Delay : UnitDelay  SampleTime=-1  HasFrameUpgradeWarning=on
  Unit Delay1 : UnitDelay  SampleTime=-1  HasFrameUpgradeWarning=on
  v1 : Outport
  v2 : Outport  Port=2
  wires:
  v0/1 -> Sum/2
  Unit Delay/1 -> Sum1/1, Sum/1  "v1(k"
  Unit Delay1/1 -> Sum2/1, MATLAB Function/2(v1), Gain/1  "v2(k)"
  Gain/1 -> Sum1/2
  Sum1/1 -> v1/1, Unit Delay/1  "v1(k+1)"
  Gain1/1 -> Sum2/2
  Sum2/1 -> v2/1, Unit Delay1/1  "v2(k+1)"
  MATLAB Function/1(y) -> Gain1/1
  Constant/1 -> MATLAB Function/3(r)
  Sum/1 -> MATLAB Function/1(delta)

== matlab function Quadrotor/Attitude Loop(LADRC)/LADRC/TD/MATLAB Function ==
  data: delta input; y output; v1 input; r input
function y = lfst(delta,v1,r)
    y = -(r*r*delta+2*r*v1);
end

== matlab function Quadrotor/Demand_LADRC/generate/butterfly/MATLAB Function ==
  data: t input; x output
function x = fcn(t)
x=cos(0.005*pi*t)*cos(0.0025*pi*t);

== matlab function Quadrotor/Demand_LADRC/generate/butterfly/MATLAB Function1 ==
  data: t input; y output
function y = fcn(t)
y=cos(0.005*pi*t)*sin(0.0025*pi*t);

== matlab function Quadrotor/Attitude Loop(LADRC)/P&R/Roll_LADRC/TD/MATLAB Function ==
  data: delta input; y output; v1 input; r input
function y = lfst(delta,v1,r)
    y = -(r*r*delta+2*r*v1);
end

== matlab function Quadrotor/Attitude Loop(LADRC)/yaw/Yaw_LADRC/TD/MATLAB Function ==
  data: delta input; y output; v1 input; r input
function y = lfst(delta,v1,r)
    y = -(r*r*delta+2*r*v1);
end

== matlab function Quadrotor/Demand_PID/generate/butterfly/MATLAB Function ==
  data: t input; x output
function x = fcn(t)
x=cos(0.005*pi*t)*cos(0.0025*pi*t);

== matlab function Quadrotor/Demand_PID/generate/butterfly/MATLAB Function1 ==
  data: t input; y output
function y = fcn(t)
y=cos(0.005*pi*t)*sin(0.0025*pi*t);

== matlab function Quadrotor/Attitude Loop(LADRC)/P&R/Pitch_LADRC/TD/MATLAB Function ==
  data: delta input; y output; v1 input; r input
function y = lfst(delta,v1,r)
    y = -(r*r*delta+2*r*v1);
end
